simulink model "sldvdemo_thrustrvs_verification_int_original"  (R2020a)
settings: Solver=FixedStepDiscrete  StartTime=0.0  StopTime=10.0  FixedStep=.1  RelTol=1e-3  EnableMultiTasking=on
PreLoadFcn:
  | load sldvdemo_thrust_reverse_bus.mat
undefined symbols (not defined in the file or in its folder): sldvsubsys
libraries: simulink x8, sldvlib x4
Description:
  | Property Proving Workflow for Thrust Reverser
settings Model: Creator=The MathWorks, Inc.  LastModifiedBy=patcanny
settings DataIOCC: ExternalInput=testdata  LimitDataPoints=on  SaveFormat=Array  ReturnWorkspaceOutputs=off
settings OptimizationCC: ExpressionDepthLimit=2147483647  InitFltsAndDblsToZero=on  LifeSpan=1  EfficientTunableParamExpr=on
settings DebuggingCC: UnderspecifiedInitializationDetection=Classic  MergeDetectMultiDrivingBlocksExec=none  SolverPrmCheckMsg=warning  FcnCallInpInsideContextMsg=warning  AllowSymbolicDim=off  StateNameClashWarn=warning  SFUnexpectedBacktrackingDiag=warning  SFNoUnconditionalDefaultTransitionDiag=warning  SFExecutionAtInitializationDiag=none  ArithmeticOperatorsInVariantConditions=warning
settings HardwareCC: ProdBitPerPointer=32  ProdBitPerSizeT=32  ProdBitPerPtrDiffT=32  ProdLargestAtomicFloat=None  ProdIntDivRoundTo=Undefined  ProdEndianess=Unspecified  ProdWordSize=32  ProdHWDeviceType=32-bit Generic
settings ModelReferenceCC: PropagateSignalLabelsOutOfModel=off
settings SFSimCC: SimUseLocalCustomCode=off  SimParseCustomCode=off  MATLABDynamicMemAlloc=off  CustomCodeUndefinedFunction=UseInterfaceOnly
settings RTWCC: Description=Real-Time Workshop Embedded Coder (no auto configuration)  SystemTargetFile=ert.tlc  GenCodeOnly=on  TemplateMakefile=ert_default_tmf  RTWUseLocalCustomCode=off
settings CodeAppCC: IgnoreCustomStorageClasses=off  CustomSymbolStrType=$N$R$M  CustomSymbolStrModelFcn=$N  StateflowObjectComments=on  InternalIdentifier=Classic
settings ERTTargetCC: MultiwordLength=2048  GenerateSampleERTMain=on  ERTCustomFileTemplate=example_file_process.tlc  ConvertIfToSwitch=off  SuppressUnreachableDefaultCases=off
settings ConfigComp: DVMode=PropertyProving  DVMaxProcessTime=900  DVUseParallel=on  DVParameters=on  DVModelCoverageObjectives=MCDC  DVMaxTestCaseSteps=500  DVTestSuiteOptimization=Auto  DVDetectActiveLogic=on  DVRebuildModelRepresentation=Always

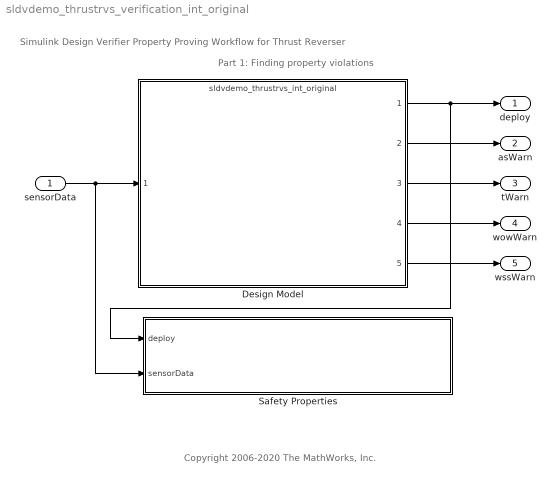
== system sldvdemo_thrustrvs_verification_int_original ==
  note: Simulink Design Verifier Property Proving Workflow for Thrust Reverser
  note: Copyright 2006-2020 The MathWorks, Inc.
  note: Part 1: Finding property violations
  sensorData : Inport  OutDataTypeStr=Bus: sldvThrustReverseBus  PortDimensions=1
  Design Model : ModelReference  ModelNameDialog=sldvdemo_thrustrvs_int_original.slx  SimulationMode=Normal  ModelReferenceVersion=1.92
  Safety Properties : Subsystem  Tag=VerificationSubsystem  DisableCoverage=on  LoadFcn=sldvsubsys('check')  TreatAsAtomicUnit=on  SimViewingDevice=on  mask(VerificationSubsystem){}
      mask init:
      | sldvsubsys('maskInit');
      settings: CopyFcn=sldvsubsys('copy');  OpenFcn=open_system(gcb,'force');
      settings: PreSaveFcn=|
      | set_param(gcb,'SimViewingDevice','on');
      | sldvsubsys('check');
      mask Help: helpview(fullfile(docroot,'toolbox','sldv','sldv.map'),'verificationsubsystem')
      mask Display: image(imread('sldvicon_versubsys.png','BackGroundColor',[1 1 1]),'center');
  deploy : Outport  OutDataTypeStr=boolean  PortDimensions=1  VectorParamsAs1DForOutWhenUnconnected=off
  asWarn : Outport  Port=2  OutDataTypeStr=boolean  PortDimensions=1  VectorParamsAs1DForOutWhenUnconnected=off
  tWarn : Outport  Port=3  OutDataTypeStr=boolean  PortDimensions=1  VectorParamsAs1DForOutWhenUnconnected=off
  wowWarn : Outport  Port=4  OutDataTypeStr=boolean  PortDimensions=1  VectorParamsAs1DForOutWhenUnconnected=off
  wssWarn : Outport  Port=5  OutDataTypeStr=boolean  PortDimensions=1  VectorParamsAs1DForOutWhenUnconnected=off
  wires:
  sensorData/1 -> Design Model/1, Safety Properties/2(sensorData)
  Design Model/1 -> deploy/1, Safety Properties/1(deploy)
  Design Model/2 -> asWarn/1
  Design Model/3 -> tWarn/1
  Design Model/4 -> wowWarn/1
  Design Model/5 -> wssWarn/1

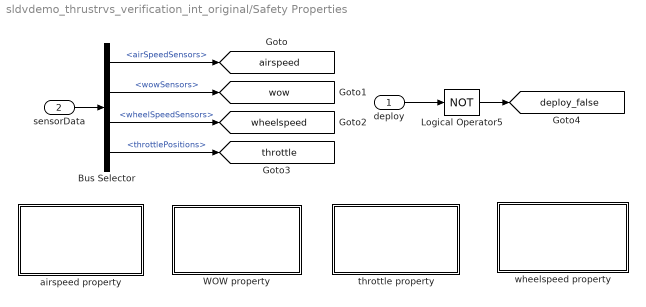
== system sldvdemo_thrustrvs_verification_int_original/Safety Properties ==
  deploy : Inport
  sensorData : Inport  Port=2
  Bus Selector : BusSelector  OutputSignals=airSpeedSensors,wowSensors,wheelSpeedSensors,throttlePositions
  Logical Operator5 : Logic  Operator=NOT  Inputs=1  AllPortsSameDT=off  OutDataTypeStr=boolean
  WOW property : Subsystem
  airspeed property : Subsystem
  throttle property : Subsystem
  wheelspeed property : Subsystem
  tag scope: airspeed=global, deploy_false=global, throttle=global, wheelspeed=global, wow=global
  wires:
  Logical Operator5/1 -> [deploy_false]
  deploy/1 -> Logical Operator5/1
  sensorData/1 -> Bus Selector/1
  Bus Selector/4 -> [throttle]  "<throttlePositions>"
  Bus Selector/3 -> [wheelspeed]  "<wheelSpeedSensors>"
  Bus Selector/2 -> [wow]  "<wowSensors>"
  Bus Selector/1 -> [airspeed]  "<airSpeedSensors>"

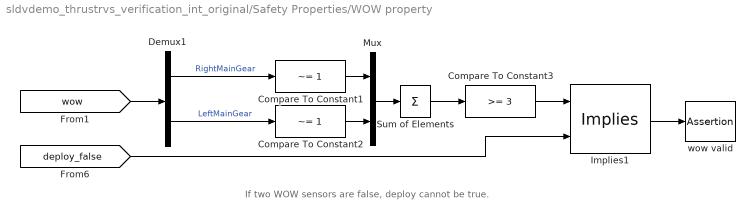
== system sldvdemo_thrustrvs_verification_int_original/Safety Properties/WOW property ==
  note: If two WOW sensors are false, deploy cannot be true.
  Compare To Constant1 : simulink/Logic and Bit Operations/Compare To Constant  relop=~=  const=1  OutDataTypeStr=uint8  ZeroCross=off
  Compare To Constant2 : simulink/Logic and Bit Operations/Compare To Constant  relop=~=  const=1  OutDataTypeStr=uint8  ZeroCross=off
  Compare To Constant3 : simulink/Logic and Bit Operations/Compare To Constant  relop=>=  const=3  OutDataTypeStr=uint8  ZeroCross=off
  Demux1 : Demux  Outputs=[2 2]
  Implies1 : sldvlib/Verification Utilities/Implies
      settings: SourceProductBaseCode=SL
  Mux : Mux  Inputs=2
  Sum of Elements : Sum  Inputs=1
  wow valid : Assertion
  wires:
  Compare To Constant3/1 -> Implies1/1
  Implies1/1 -> wow valid/1
  [wow] -> Demux1/1
  [deploy_false] -> Implies1/2
  Mux/1 -> Sum of Elements/1
  Compare To Constant2/1 -> Mux/2
  Compare To Constant1/1 -> Mux/1
  Sum of Elements/1 -> Compare To Constant3/1
  Demux1/2 -> Compare To Constant2/1  "LeftMainGear"
  Demux1/1 -> Compare To Constant1/1  "RightMainGear"

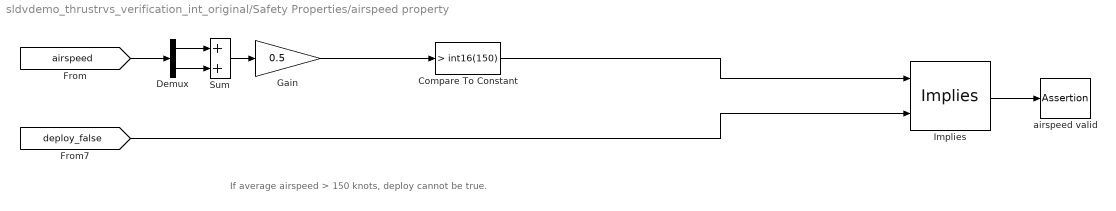
== system sldvdemo_thrustrvs_verification_int_original/Safety Properties/airspeed property ==
  note: If average airspeed > 150 knots, deploy cannot be true.
  Compare To Constant : simulink/Logic and Bit Operations/Compare To Constant  relop=>  const=int16(150)  OutDataTypeStr=uint8  ZeroCross=off
  Demux : Demux  Outputs=2
  Gain : Gain  Gain=0.5
  Implies : sldvlib/Verification Utilities/Implies
      settings: SourceProductBaseCode=SL
  Sum : Sum
  airspeed valid : Assertion
  wires:
  [deploy_false] -> Implies/2
  Implies/1 -> airspeed valid/1
  [airspeed] -> Demux/1
  Sum/1 -> Gain/1
  Demux/2 -> Sum/2
  Demux/1 -> Sum/1
  Gain/1 -> Compare To Constant/1
  Compare To Constant/1 -> Implies/1

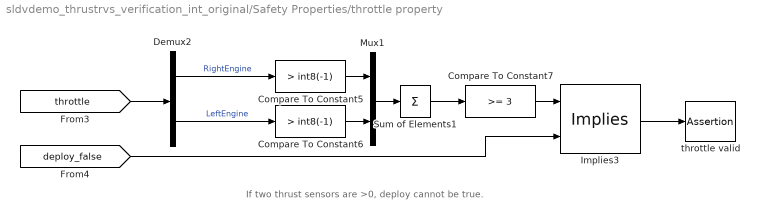
== system sldvdemo_thrustrvs_verification_int_original/Safety Properties/throttle property ==
  note: If two thrust sensors are >0, deploy cannot be true.
  Compare To Constant5 : simulink/Logic and Bit Operations/Compare To Constant  relop=>  const=int8(-1)  OutDataTypeStr=uint8  ZeroCross=off
  Compare To Constant6 : simulink/Logic and Bit Operations/Compare To Constant  relop=>  const=int8(-1)  OutDataTypeStr=uint8  ZeroCross=off
  Compare To Constant7 : simulink/Logic and Bit Operations/Compare To Constant  relop=>=  const=3  OutDataTypeStr=uint8  ZeroCross=off
  Demux2 : Demux  Outputs=[2 2]
  Implies3 : sldvlib/Verification Utilities/Implies
      settings: SourceProductBaseCode=SL
  Mux1 : Mux  Inputs=2
  Sum of Elements1 : Sum  Inputs=1
  throttle valid : Assertion
  wires:
  Implies3/1 -> throttle valid/1
  [deploy_false] -> Implies3/2
  Compare To Constant7/1 -> Implies3/1
  [throttle] -> Demux2/1
  Mux1/1 -> Sum of Elements1/1
  Compare To Constant6/1 -> Mux1/2
  Compare To Constant5/1 -> Mux1/1
  Sum of Elements1/1 -> Compare To Constant7/1
  Demux2/2 -> Compare To Constant6/1  "LeftEngine"
  Demux2/1 -> Compare To Constant5/1  "RightEngine"

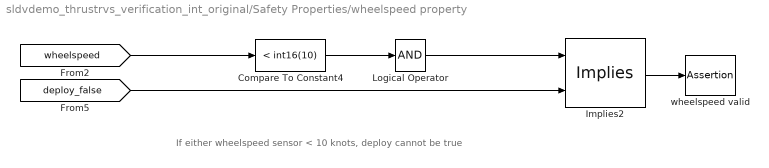
== system sldvdemo_thrustrvs_verification_int_original/Safety Properties/wheelspeed property ==
  note: If either wheelspeed sensor < 10 knots, deploy cannot be true
  Compare To Constant4 : simulink/Logic and Bit Operations/Compare To Constant  relop=<  const=int16(10)  OutDataTypeStr=uint8  ZeroCross=off
  Implies2 : sldvlib/Verification Utilities/Implies
      settings: SourceProductBaseCode=SL
  Logical Operator : Logic  Inputs=1  AllPortsSameDT=off  OutDataTypeStr=boolean
  wheelspeed valid : Assertion
  wires:
  Implies2/1 -> wheelspeed valid/1
  [deploy_false] -> Implies2/2
  Logical Operator/1 -> Implies2/1
  Compare To Constant4/1 -> Logical Operator/1
  [wheelspeed] -> Compare To Constant4/1
